simulink model "pvt_tegs_vienna"  (R2023b)
settings: Solver=ode14x  StartTime=0.0  StopTime=3*24*3600  FixedStep=1  RelTol=1e-06
PreLoadFcn:
  | sscv_hybrid_solar_panel_data
values from neighbouring files (symbols this model uses):
  Inclination = struct()    [meteo_data_struct.m]
  Irradiance_si = struct()    [meteo_data_struct.m]
  Irradiance_ts = struct()    [meteo_data_struct.m]
  load = struct()    [pvt_tegs_data.m]
  month = months{m}    [AUTOMATICO_mix.m]    (also in AUTOMATICO_parallel.m; AUTOMATICO_series.m)
  panel = struct()    [pvt_tegs_data.m]
  pipe = struct()    [pvt_tegs_data.m]
  pumps = struct()    [pvt_tegs_data.m]
  T_ext = struct()    [meteo_data_struct.m]
  tank = struct()    [pvt_tegs_data.m]
  teg = struct()    [pvt_tegs_data.m]
libraries: fl_lib x69, nesl_utility x35, simulink x5, ee_lib x2, My_second_lib x1, SimscapeFluids_lib x1
(part 2 of 2)

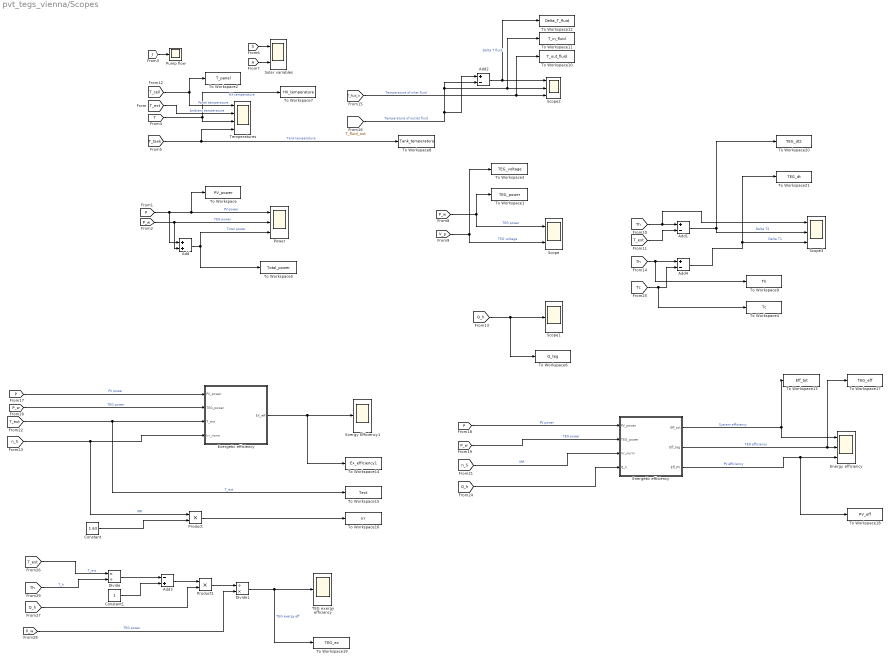
== system pvt_tegs_vienna/Scopes ==
  Add : Sum
  Add1 : Sum  Inputs=+-
  Add2 : Sum  Inputs=+-
  Add3 : Sum  Inputs=-+
  Add4 : Sum  Inputs=+-
  Constant : Constant  Value=1.63
  Constant1 : Constant
  Divide : Product  Inputs=*/
  Divide1 : Product  Inputs=/*
  Energetic efficiency : MATLAB Function  TreatAsAtomicUnit=on
  Energy efficiency : Scope  NumInputPorts=3
  Exergetic efficiency : MATLAB Function  TreatAsAtomicUnit=on
  Exergy Efficiency1 : Scope
  From7 : From  TagVisibility=global
  Power : Scope  NumInputPorts=3
  Product : Product
  Product1 : Product
  Pump flow : Scope
  Scope : Scope  NumInputPorts=2
  Scope1 : Scope
  Scope2 : Scope  NumInputPorts=3
  Scope3 : Scope  NumInputPorts=3
  Solar variables : Scope  NumInputPorts=2
  TEG exergy efficiency : Scope
  Temperatures : Scope  NumInputPorts=4
  To Workspace : ToWorkspace  VariableName=PV_power  SaveFormat=Structure With Time  SampleTime=-1
  To Workspace1 : ToWorkspace  VariableName=TEG_power  SaveFormat=Structure With Time  SampleTime=-1
  To Workspace10 : ToWorkspace  VariableName=T_out_fluid  SaveFormat=Structure With Time  SampleTime=-1
  To Workspace11 : ToWorkspace  VariableName=T_in_fluid  SaveFormat=Structure With Time  SampleTime=-1
  To Workspace12 : ToWorkspace  VariableName=Delta_T_fluid  SaveFormat=Structure With Time  SampleTime=-1
  To Workspace13 : ToWorkspace  VariableName=Eff_tot  SaveFormat=Structure With Time  SampleTime=-1
  To Workspace14 : ToWorkspace  VariableName=Ex_efficiency1  SaveFormat=Structure With Time  SampleTime=-1
  To Workspace15 : ToWorkspace  VariableName=Text  SaveFormat=Structure With Time  SampleTime=-1
  To Workspace16 : ToWorkspace  VariableName=Irr  SaveFormat=Structure With Time  SampleTime=-1
  To Workspace17 : ToWorkspace  VariableName=TEG_eff  SaveFormat=Structure With Time  SampleTime=-1
  To Workspace18 : ToWorkspace  VariableName=PV_eff  SaveFormat=Structure With Time  SampleTime=-1
  To Workspace19 : ToWorkspace  VariableName=TEG_ex  SaveFormat=Structure With Time  SampleTime=-1
  To Workspace2 : ToWorkspace  VariableName=T_panel  SaveFormat=Structure With Time  SampleTime=-1
  To Workspace20 : ToWorkspace  VariableName=TEG_dt2  SaveFormat=Structure With Time  SampleTime=-1
  To Workspace21 : ToWorkspace  VariableName=TEG_dt  SaveFormat=Structure With Time  SampleTime=-1
  To Workspace3 : ToWorkspace  VariableName=TEG_voltage  SaveFormat=Structure With Time  SampleTime=-1
  To Workspace4 : ToWorkspace  VariableName=Tc  SaveFormat=Structure With Time  SampleTime=-1
  To Workspace5 : ToWorkspace  VariableName=Total_power  SaveFormat=Structure With Time  SampleTime=-1
  To Workspace6 : ToWorkspace  VariableName=Q_teg  SaveFormat=Structure With Time  SampleTime=-1
  To Workspace7 : ToWorkspace  VariableName=HX_temperature  SaveFormat=Structure With Time  SampleTime=-1
  To Workspace8 : ToWorkspace  VariableName=Tank_temperature  SaveFormat=Structure With Time  SampleTime=-1
  To Workspace9 : ToWorkspace  VariableName=Th  SaveFormat=Structure With Time  SampleTime=-1
  wires:
  [P] -> Add/1, To Workspace/1, Power/1  "PV power"
  [J] -> Pump flow/1
  [S] -> Solar variables/1
  From7/1 -> Solar variables/2
  [T] -> To Workspace7/1, Temperatures/3  "HX temperature"
  [T_tank] -> Temperatures/4, To Workspace8/1  "Tank temperature"
  [T_ext] -> Temperatures/2  "Ambient temperature"
  [P_w] -> Add/2, Power/2  "TEG power"
  Add/1 -> To Workspace5/1, Power/3  "Total power"
  [P_w] -> To Workspace1/1, Scope/1  "TEG power"
  [V_p] -> To Workspace3/1, Scope/2  "TEG voltage"
  [T_cell] -> To Workspace2/1, Temperatures/1  "Panel temperature"
  [Q_h] -> To Workspace6/1, Scope1/1
  [T_fluid_out] -> Add2/1, To Workspace10/1, Scope2/3  "Temperature of outlet fluid"
  [T_fluid_in] -> To Workspace11/1, Scope2/2, Add2/2  "Temperature of inlet fluid"
  Add2/1 -> To Workspace12/1, Scope2/1  "Delta T fluid"
  [P] -> Exergetic efficiency/1(PV_power)  "PV power"
  [P_w] -> Exergetic efficiency/2(TEG_power)  "TEG power"
  [T_ext] -> To Workspace15/1, Exergetic efficiency/3(T_ext)  "T_ext"
  [n_S] -> Product/1, Exergetic efficiency/4(Irr_norm)  "IRR"
  Exergetic efficiency/1(EX_eff) -> To Workspace14/1, Exergy Efficiency1/1
  [P] -> Energetic efficiency/1(PV_power)  "PV power"
  [P_w] -> Energetic efficiency/2(TEG_power)  "TEG power"
  [n_S] -> Energetic efficiency/3(Irr_norm)  "IRR"
  [Q_h] -> Energetic efficiency/4(Q_h)
  Energetic efficiency/1(Eff_tot) -> To Workspace13/1, Energy efficiency/1  "System efficiency"
  Energetic efficiency/2(Eff_teg) -> Energy efficiency/2, To Workspace17/1  "TEG efficiency"
  Energetic efficiency/3(Eff_PV) -> To Workspace18/1, Energy efficiency/3  "PV efficiency"
  Constant/1 -> Product/2
  Product/1 -> To Workspace16/1
  [T_ext] -> Divide/1  "T_ext"
  Divide/1 -> Add3/1
  Constant1/1 -> Add3/2
  Add3/1 -> Product1/1
  [Q_h] -> Product1/2
  Product1/1 -> Divide1/1
  [P_w] -> Divide1/2  "TEG power"
  Divide1/1 -> To Workspace19/1, TEG exergy efficiency/1  "TEG exergy eff"
  [Th] -> Divide/2  "T_h"
  [Th] -> Add4/1, To Workspace9/1
  [Tc] -> To Workspace4/1, Add4/2
  Add4/1 -> To Workspace21/1, Scope3/3  "Delta T1"
  [Th] -> Scope3/1, Add1/1
  [T_ext] -> Add1/2
  Add1/1 -> To Workspace20/1, Scope3/2  "Delta T2"

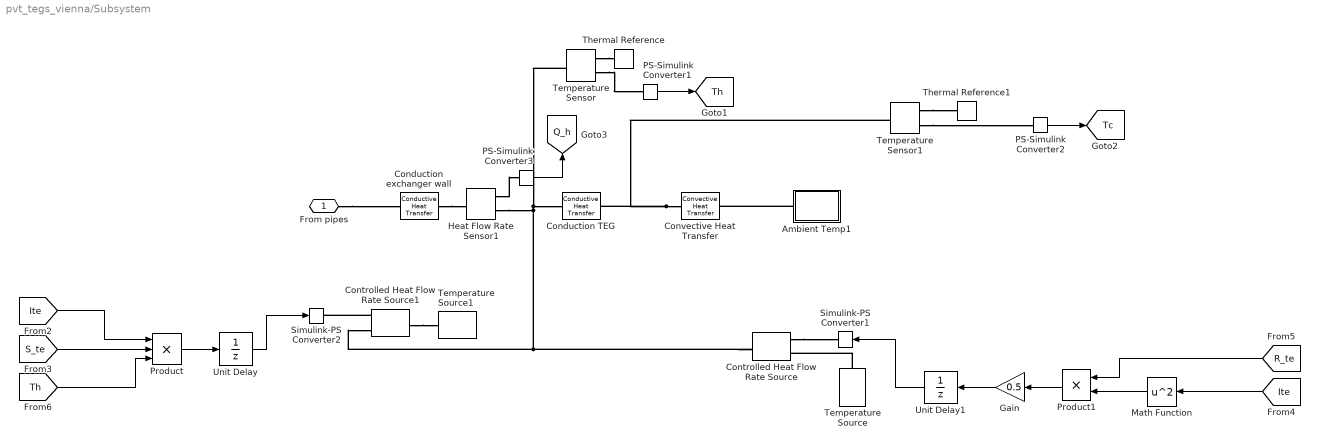
== system pvt_tegs_vienna/Subsystem ==
  Ambient Temp1 : Subsystem
  Conduction TEG : fl_lib/Thermal/Thermal Elements/Conductive Heat Transfer  thermal_type=foundation.enum.ConstantVariableTabulated.Constant  wall_geometry=foundation.enum.ConductionWallGeometry.Planar  area=teg.A_tot m^2  thickness=teg.d m  d_in=0.05 m  d_out=0.1 m  L=1 m  th_cond_min=10 W/(K*m)  th_cond=teg.l W/(m*K)  th_cond_TLU=[413, 401, 392, 383, 371, 357, 342] W/(K*m)  temp_TLU=[200, 273, 400, 600, 800, 1000, 1200] K  T_specify=off  T_priority=None  T=0 K  T_nominal_specify=off  T_nominal_unit=K  T_nominal_value=1  Q_specify=off  Q_priority=None  Q=0 W  Q_nominal_specify=off  Q_nominal_unit=W  Q_nominal_value=1
  Conduction exchanger wall : fl_lib/Thermal/Thermal Elements/Conductive Heat Transfer  thermal_type=foundation.enum.ConstantVariableTabulated.Constant  wall_geometry=foundation.enum.ConductionWallGeometry.Planar  area=teg.A_tot m^2  thickness=panel.heatTransfer.Le m  d_in=0.05 m  d_out=0.1 m  L=1 m  th_cond_min=10 W/(K*m)  th_cond=panel.heatTransfer.ke W/(m*K)  th_cond_TLU=[413, 401, 392, 383, 371, 357, 342] W/(K*m)  temp_TLU=[200, 273, 400, 600, 800, 1000, 1200] K  T_specify=off  T_priority=None  T=0 K  T_nominal_specify=off  T_nominal_unit=K  T_nominal_value=1  Q_specify=off  Q_priority=None  Q=0 W  Q_nominal_specify=off  Q_nominal_unit=W  Q_nominal_value=1
  Controlled Heat Flow Rate Source : fl_lib/Thermal/Thermal Sources/Controlled Heat Flow Rate Source
  Controlled Heat Flow Rate Source1 : fl_lib/Thermal/Thermal Sources/Controlled Heat Flow Rate Source
  Convective Heat Transfer : fl_lib/Thermal/Thermal Elements/Convective Heat Transfer  thermal_type=foundation.enum.constant_variable.constant  area=teg.A_tot m^2  heat_tr_coeff=teg.heat_conv W/(K*m^2)  min_heat_tr_coeff=1e-3 W/(K*m^2)  T_specify=off  T_priority=None  T=0 K  T_nominal_specify=off  T_nominal_unit=K  T_nominal_value=1  Q_specify=off  Q_priority=None  Q=0 W  Q_nominal_specify=off  Q_nominal_unit=W  Q_nominal_value=1
  Gain : Gain  Gain=0.5
  Heat Flow Rate Sensor1 : fl_lib/Thermal/Thermal Sensors/Heat Flow Rate Sensor
  Math Function : Math  Operator=square
  PS-Simulink Converter1 : nesl_utility/PS-Simulink Converter  PhysicalDomain=network_engine_domain  SubClassName=ps_output  LeftPortType=input  RightPortType=output  PseudoPeriodic=off  Frequencies=[]  VectorFormat=inherit  Unit=K  AffineConversion=off
  PS-Simulink Converter2 : nesl_utility/PS-Simulink Converter  PhysicalDomain=network_engine_domain  SubClassName=ps_output  LeftPortType=input  RightPortType=output  PseudoPeriodic=off  Frequencies=[]  VectorFormat=inherit  Unit=K  AffineConversion=off
  PS-Simulink Converter3 : nesl_utility/PS-Simulink Converter  PhysicalDomain=network_engine_domain  SubClassName=ps_output  LeftPortType=input  RightPortType=output  PseudoPeriodic=off  Frequencies=[]  VectorFormat=inherit  Unit=inherit  AffineConversion=off
  Product : Product  Inputs=3
  Product1 : Product
  Simulink-PS Converter1 : nesl_utility/Simulink-PS Converter  PhysicalDomain=network_engine_domain  SubClassName=ps_input  LeftPortType=input  RightPortType=output  PseudoPeriodic=off  Frequencies=[]  NoiseDistribution=none  NoiseParameters=[]  Unit=1  AffineConversion=off  FilteringAndDerivatives=provide  SimscapeFilterOrder=1  InputFilterTimeConstant=0.001  UdotUserProvided=0
  Simulink-PS Converter2 : nesl_utility/Simulink-PS Converter  PhysicalDomain=network_engine_domain  SubClassName=ps_input  LeftPortType=input  RightPortType=output  PseudoPeriodic=off  Frequencies=[]  NoiseDistribution=none  NoiseParameters=[]  Unit=1  AffineConversion=off  FilteringAndDerivatives=provide  SimscapeFilterOrder=1  InputFilterTimeConstant=0.001  UdotUserProvided=0
  Temperature Sensor : fl_lib/Thermal/Thermal Sensors/Temperature Sensor  temperature_measure=foundation.enum.MeasurementReference.difference
  Temperature Sensor1 : fl_lib/Thermal/Thermal Sensors/Temperature Sensor  temperature_measure=foundation.enum.MeasurementReference.difference
  Temperature Source : fl_lib/Thermal/Thermal Sources/Temperature Source  temperature=293.15 K
  Temperature Source1 : fl_lib/Thermal/Thermal Sources/Temperature Source  temperature=293.15 K
  Thermal Reference : fl_lib/Thermal/Thermal Elements/Thermal Reference
  Thermal Reference1 : fl_lib/Thermal/Thermal Elements/Thermal Reference
  Unit Delay : UnitDelay  SampleTime=-1  HasFrameUpgradeWarning=on
  Unit Delay1 : UnitDelay  SampleTime=-1  HasFrameUpgradeWarning=on
  From pipes : PMIOPort  Side=Right
  tag scope: Q_h=global, Tc=global, Th=global
  wires:
  PS-Simulink Converter1/1 -> [Th]
  [Ite] -> Math Function/1
  Math Function/1 -> Product1/2
  Product1/1 -> Gain/1
  [R_te] -> Product1/1
  [Ite] -> Product/1
  [S_te] -> Product/2
  Product/1 -> Unit Delay/1
  PS-Simulink Converter2/1 -> [Tc]
  [Th] -> Product/3
  Gain/1 -> Unit Delay1/1
  Unit Delay1/1 -> Simulink-PS Converter1/1
  Unit Delay/1 -> Simulink-PS Converter2/1
  PS-Simulink Converter3/1 -> [Q_h]
  connections:
  From pipes/RConn1 -- Conduction exchanger wall/LConn1
  Convective Heat Transfer/LConn1 -- Temperature Sensor1/LConn1 -- Conduction TEG/RConn1
  Ambient Temp1/LConn1 -- Convective Heat Transfer/RConn1
  Controlled Heat Flow Rate Source/LConn1 -- Temperature Sensor/LConn1 -- Conduction TEG/LConn1 -- Heat Flow Rate Sensor1/RConn2 -- Controlled Heat Flow Rate Source1/RConn2
  Temperature Sensor/RConn2 -- PS-Simulink Converter1/LConn1
  Temperature Sensor/RConn1 -- Thermal Reference/LConn1
  Temperature Source/LConn1 -- Controlled Heat Flow Rate Source/RConn2
  Controlled Heat Flow Rate Source/RConn1 -- Simulink-PS Converter1/RConn1
  Controlled Heat Flow Rate Source1/LConn1 -- Temperature Source1/LConn1
  Controlled Heat Flow Rate Source1/RConn1 -- Simulink-PS Converter2/RConn1
  Temperature Sensor1/RConn1 -- Thermal Reference1/LConn1
  Temperature Sensor1/RConn2 -- PS-Simulink Converter2/LConn1
  Conduction exchanger wall/RConn1 -- Heat Flow Rate Sensor1/LConn1
  Heat Flow Rate Sensor1/RConn1 -- PS-Simulink Converter3/LConn1

== system pvt_tegs_vienna/T sensor ==
  PS-Simulink Converter2 : nesl_utility/PS-Simulink Converter  PhysicalDomain=network_engine_domain  SubClassName=ps_output  LeftPortType=input  RightPortType=output  PseudoPeriodic=off  Frequencies=[]  VectorFormat=1-D array  Unit=K  AffineConversion=off
  Temperature Sensor : fl_lib/Thermal/Thermal Sensors/Temperature Sensor  temperature_measure=foundation.enum.MeasurementReference.difference
  Thermal Reference : fl_lib/Thermal/Thermal Elements/Thermal Reference
  A : PMIOPort  Side=Left
  tag scope: T=global
  wires:
  PS-Simulink Converter2/1 -> [T]
  connections:
  Temperature Sensor/LConn1 -- A/RConn1
  Thermal Reference/LConn1 -- Temperature Sensor/RConn1
  PS-Simulink Converter2/LConn1 -- Temperature Sensor/RConn2

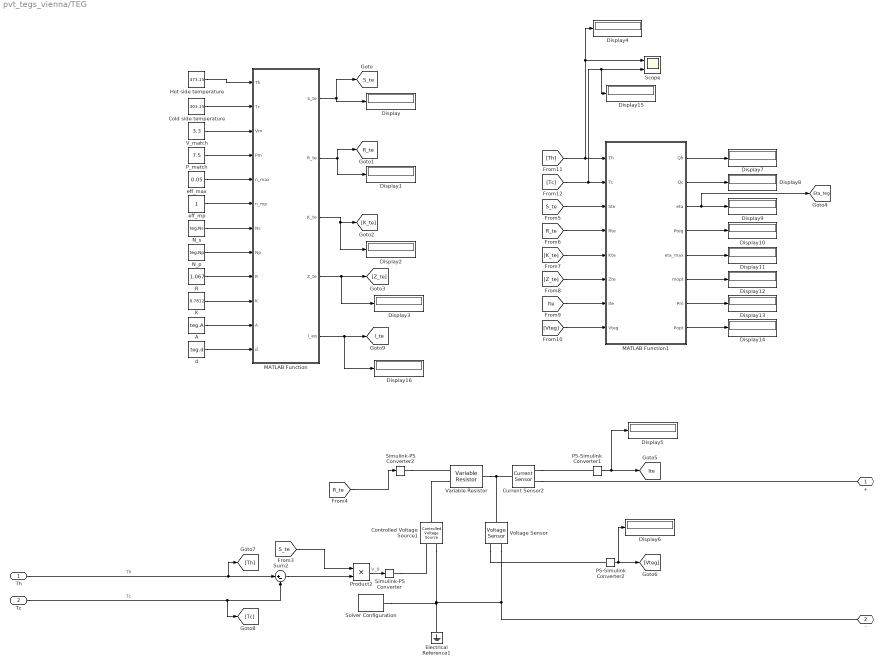
== system pvt_tegs_vienna/TEG ==
  Th : Inport
  Tc : Inport  Port=2
  A : Constant  Value=teg.A
  Cold side temperature : Constant  Value=303.15
  Controlled Voltage Source1 : fl_lib/Electrical/Electrical Sources/Controlled Voltage Source
  Current Sensor2 : fl_lib/Electrical/Electrical Sensors/Current Sensor
  Display{,1..16} (17 alike) : Display
  Electrical Reference1 : fl_lib/Electrical/Electrical Elements/Electrical Reference
  Hot side temperature : Constant  Value=473.15
  K : Constant  Value=0.7812
  MATLAB Function : MATLAB Function  TreatAsAtomicUnit=on
  MATLAB Function1 : MATLAB Function  TreatAsAtomicUnit=on
  N_p : Constant  Value=teg.Np
  N_s : Constant  Value=teg.Ns
  PS-Simulink Converter1 : nesl_utility/PS-Simulink Converter  PhysicalDomain=network_engine_domain  SubClassName=ps_output  LeftPortType=input  RightPortType=output  PseudoPeriodic=off  Frequencies=[]  VectorFormat=inherit  Unit=inherit  AffineConversion=off
  PS-Simulink Converter2 : nesl_utility/PS-Simulink Converter  PhysicalDomain=network_engine_domain  SubClassName=ps_output  LeftPortType=input  RightPortType=output  PseudoPeriodic=off  Frequencies=[]  VectorFormat=inherit  Unit=inherit  AffineConversion=off
  P_match : Constant  Value=7.5
  Product2 : Product
  R : Constant  Value=1.067
  Scope : Scope  NumInputPorts=2
  Simulink-PS Converter : nesl_utility/Simulink-PS Converter  PhysicalDomain=network_engine_domain  SubClassName=ps_input  LeftPortType=input  RightPortType=output  PseudoPeriodic=off  Frequencies=[]  NoiseDistribution=none  NoiseParameters=[]  Unit=1  AffineConversion=off  FilteringAndDerivatives=provide  SimscapeFilterOrder=1  InputFilterTimeConstant=0.001  UdotUserProvided=0
  Simulink-PS Converter2 : nesl_utility/Simulink-PS Converter  PhysicalDomain=network_engine_domain  SubClassName=ps_input  LeftPortType=input  RightPortType=output  PseudoPeriodic=off  Frequencies=[]  NoiseDistribution=none  NoiseParameters=[]  Unit=1  AffineConversion=off  FilteringAndDerivatives=provide  SimscapeFilterOrder=1  InputFilterTimeConstant=0.001  UdotUserProvided=0
  Solver Configuration : nesl_utility/Solver Configuration  PhysicalDomain=network_engine_domain  SubClassName=solver  LeftPortType=input  RightPortType=generic  Tones=[]  Harmonics=[]  SimulateNoise=off  Profile=off  UseLocalSampling=off  EnableSwitchedLinearOptims=on  FrequencyDomain=off  UseCCode=off  RelTol=0.001  AbsTol=0.001  MinStep=1e-09  ToWorkspace=off  RevertToSquareIcSolve=off  NumHomotopyIterations=100  PhasorMode=off  PhasorModeNumHarmonics=1  ConsistencySolver=NEWTON_XTOL_AFTER_FTOL  IndexReductionMethod=DerivativeReplacement  DoDC=off  ResidualTolerance=1e-09  ConsistencyTolSource=GLOBAL  ConsistencyAbsTol=0.001  ConsistencyRelTol=0.001  ConsistencyTolFactor=0.001  UseLocalSolver=off  LocalSolverChoice=NE_BACKWARD_EULER_ADVANCER  ResolveIndetEquations=on  FunctionEvalNumThread=1  LocalSolverSampleTime=0.001  DoFixedCost=off  MaxNonlinIter=3  MaxModeIter=2  ComputeImpulses=off  ImpulseIterations=2  LinearAlgebra=auto  LinearAlgebraNumThread=0  EquationFormulation=NE_TIME_EF  DelaysMemoryBudget=1024  AutomaticFiltering=on  FilteringTimeConstant=0.001  PartitionStorageMethod=AS_NEEDED  PartitionMemoryBudget=1024  PartitionMethod=ROBUST  MultibodyUseLocalSolver=off  MultibodyLocalSolverChoice=ODE1  MultibodyLocalSolverSampleTime=0.001
  Sum2 : Sum  Inputs=|+-
  V_match : Constant  Value=3.3
  Variable Resistor : fl_lib/Electrical/Electrical Elements/Variable Resistor  Rmin=0 Ohm  thermalEnable=false  thermal_mass=1 J/K  i_specify=off  i_priority=None  i=0 A  i_nominal_specify=off  i_nominal_unit=A  i_nominal_value=1  v_specify=off  v_priority=None  v=0 V  v_nominal_specify=off  v_nominal_unit=V  v_nominal_value=1  T_specify=off  T_priority=None  T=300 K  T_nominal_specify=off  T_nominal_unit=K  T_nominal_value=1
  Voltage Sensor : fl_lib/Electrical/Electrical Sensors/Voltage Sensor
  d : Constant  Value=teg.d
  eff_max : Constant  Value=0.05
  eff_mp : Constant
  + : PMIOPort  Side=Right
  - : PMIOPort  Port=2  Side=Right
  tag scope: Eta_teg=global, Ite=global, R_te=global, S_te=global, l_te=global
  wires:
  Th/1 -> [Th], Sum2/1  "Th"
  MATLAB Function/4(Z_te) -> Display3/1, [Z_te]
  [Z_te] -> MATLAB Function1/6(Zte)
  N_p/1 -> MATLAB Function/8(Np)
  eff_mp/1 -> MATLAB Function/6(n_mp)
  MATLAB Function/2(R_te) -> Display1/1, [R_te]
  eff_max/1 -> MATLAB Function/5(n_max)
  P_match/1 -> MATLAB Function/4(Pm)
  [Th] -> Display4/1, Scope/1, MATLAB Function1/1(Th)
  PS-Simulink Converter1/1 -> [Ite], Display5/1
  MATLAB Function1/1(Qh) -> Display7/1
  MATLAB Function/3(K_te) -> Display2/1, [K_te]
  [K_te] -> MATLAB Function1/5(Kte)
  PS-Simulink Converter2/1 -> Display6/1, [Vteg]
  MATLAB Function1/7(Pm) -> Display13/1
  Cold side temperature/1 -> MATLAB Function/2(Tc)
  MATLAB Function1/3(eta) -> [Eta_teg], Display9/1
  Tc/1 -> [Tc], Sum2/2  "Tc"
  Hot side temperature/1 -> MATLAB Function/1(Th)
  MATLAB Function/1(S_te) -> Display/1, [S_te]
  MATLAB Function1/6(mopt) -> Display12/1
  V_match/1 -> MATLAB Function/3(Vm)
  Product2/1 -> Simulink-PS Converter/1  "V_0"
  [S_te] -> Product2/1
  MATLAB Function1/4(Pteg) -> Display10/1
  N_s/1 -> MATLAB Function/7(Ns)
  [S_te] -> MATLAB Function1/3(Ste)
  MATLAB Function1/8(Popt) -> Display14/1
  MATLAB Function1/2(Qc) -> Display8/1
  [R_te] -> Simulink-PS Converter2/1
  MATLAB Function1/5(eta_max) -> Display11/1
  [Vteg] -> MATLAB Function1/8(Vteg)
  Sum2/1 -> Product2/2
  [R_te] -> MATLAB Function1/4(Rte)
  [Ite] -> MATLAB Function1/7(Ite)
  R/1 -> MATLAB Function/9(R)
  K/1 -> MATLAB Function/10(K)
  A/1 -> MATLAB Function/11(A)
  d/1 -> MATLAB Function/12(d)
  MATLAB Function/5(l_eq) -> Display16/1, [l_te]
  [Tc] -> Display15/1, Scope/2, MATLAB Function1/2(Tc)
  connections:
  Variable Resistor/RConn1 -- Voltage Sensor/LConn1 -- Current Sensor2/LConn1
  Current Sensor2/RConn2 -- +/RConn1
  Current Sensor2/RConn1 -- PS-Simulink Converter1/LConn1
  Controlled Voltage Source1/RConn2 -- Solver Configuration/RConn1 -- Electrical Reference1/LConn1 -- -/RConn1 -- Voltage Sensor/RConn2
  Controlled Voltage Source1/LConn1 -- Variable Resistor/LConn2
  Simulink-PS Converter/RConn1 -- Controlled Voltage Source1/RConn1
  Simulink-PS Converter2/RConn1 -- Variable Resistor/LConn1
  Voltage Sensor/RConn1 -- PS-Simulink Converter2/LConn1

== system pvt_tegs_vienna/Subsystem/Ambient Temp1 ==
  Controlled Temperature Source : fl_lib/Thermal/Thermal Sources/Controlled Temperature Source
  Simulink-PS Converter1 : nesl_utility/Simulink-PS Converter  PhysicalDomain=network_engine_domain  SubClassName=ps_input  LeftPortType=input  RightPortType=output  PseudoPeriodic=off  Frequencies=[]  NoiseDistribution=none  NoiseParameters=[]  Unit=K  AffineConversion=off  FilteringAndDerivatives=provide  SimscapeFilterOrder=1  InputFilterTimeConstant=0.001  UdotUserProvided=0
  Thermal Reference1 : fl_lib/Thermal/Thermal Elements/Thermal Reference
  Conn1 : PMIOPort  Side=Left
  wires:
  [T_ext] -> Simulink-PS Converter1/1
  connections:
  Controlled Temperature Source/LConn1 -- Conn1/RConn1
  Thermal Reference1/LConn1 -- Controlled Temperature Source/RConn2
  Simulink-PS Converter1/RConn1 -- Controlled Temperature Source/RConn1

== matlab function pvt_tegs_vienna/TEG/MATLAB Function ==
  data: Th input; S_te output; Tc input; Vm input; Pm input; n_max input; n_mp input; Ns input; Np input; R_te output; K_te output; Z_te output; R input; K input; l_eq output; A input; d input
function [S_te, R_te, K_te, Z_te, l_eq] = Teg_properties(Th,Tc,Vm,Pm,n_max,n_mp,Ns,Np,R,K,A,d)

%MODULE:
%Th: hot side temperature at which TEG properties are measured
%Tc: cold side temperature at which TEG properties are measured
%Vm: matched load voltage of module (maximum power at given DT)
%Pm: matched power (maximum power at given DT)
%n_max: maximum efficiency of TEG at given DT
%n_mp: matched efficiency (efficiency of TEG at maximum power point g.DT)
%A: area of the module [m^2]
%d: thickness of the module [m]

%CONNECTION:
%Ns: number of series-connected TEGs modules
%Np: number of electrically parallel connected groups of modules. 

%Temperature difference
D_T=Th-Tc;

%Average temperature
T_avr=(Th+Tc)/2;

%Seebeck coefficient of module
Sm=2*Vm/D_T;

%Internal resistance of module
if isnan(R) 
    Rm=Vm^2/Pm;
else
    Rm=R;
end

%Conduttance of the module
if isnan(K)
    Km=(Sm^2*(D_T-n_max*Th)^2)/(2*(2-n_max)*D_T*n_max*Rm);
else
    Km=K;
end

%Km=(Sm^2*(D_T-n_mp*(Th+T_avr)))/(4*n_mp*Rm)


%Figure of merit of module
Zm=Sm^2/(Rm*Km);

%Converting the parameters for 1 module to Ns, Np modules
S_te=Ns*Sm;
R_te=(Ns/Np)*Rm;
K_te=Ns*Np*Km;
Z_te=Zm;
l_eq=(d*K_te)/A;
end

== matlab function pvt_tegs_vienna/Optical model/MATLAB Function ==
  data: S input; Ir output; Incl input; heatg output; powAbspv output; panel parameter
function [Ir, heatg, powAbspv] = optics(S, Incl, panel)
    
    %This function computes the reflection, absorption and transmission in
    %the glass to compute the irradiation to the PV cells, the heat absorbed 
    %in the glass and the radiation power absorbed in the PV cells,
    %it is based on Fresnel's laws, depending on the incident angle
    
    Ncell = panel.geometry.Ncell;
    Acell = panel.geometry.Acell;
    Apanel = panel.geometry.Apanel;
    ng = panel.optical.ng;
    absg = panel.optical.absg;
    dg = panel.optical.dg;
    rpv = panel.optical.rpv;
   

    % Fresnel equations 1st boundary
    r1p =  ( ng^2*cos(Incl) - sqrt(ng^2 - sin(Incl)^2) )^2/( ng^2*cos(Incl) + sqrt( ng^2 - sin(Incl)^2 ) )^2; %P polarization
    r1s =  ( cos(Incl) - sqrt(ng^2 - sin(Incl)^2) )^2/( cos(Incl) + sqrt( ng^2 - sin(Incl)^2 ) )^2; %S polarization
    r1 = 0.5*(r1p + r1s); %Effective reflectance
    t1 = 1-r1;

    nga = 1/ng; %refractive index glass -> air
    th2 = asin(sin(Incl)/ng);  %Snell's law to compute angle of incidence on 2nd boundary

    % Fresnel equations 2nd boundary
    r2p = ( nga^2*cos(th2) - sqrt(nga^2 - sin(th2)^2) )^2/( nga^2*cos(th2) + sqrt( nga^2 - sin(th2)^2 ) )^2 ;
    r2s = ( cos(th2) - sqrt(nga^2 - sin(th2)^2) )^2/( cos(th2) + sqrt( nga^2 - sin(th2)^2 ) )^2 ;
    r2 = 0.5*(r2p + r2s); %Effective reflectance
    t2 = 1 - r2;

    taug = exp(-absg*dg/cos(th2)); 
    
    %Total coefficients for infinite reflections between 2 parallel boundaries
    Transg = t1*taug*t2/(1 - r1*r2*taug^2);
    Reflg = r1 + (t1^2*taug^2*r2)/(1 - r1*r2*taug^2);
    Absg = 1 - Transg - Reflg; 

    Ir = S*Transg; %Irradiation to the PV cells
    heatg = Apanel*Absg*S; %heat absorbed in the glass
    powAbspv = Apanel*Transg*(1-rpv)*S; %radiation power absorbed by PV cells. Part of it transforms in electrical power
    
end

== matlab function pvt_tegs_vienna/TEG/MATLAB Function1 ==
  data: Th input; Qh output; Tc input; Ste input; Rte input; Kte input; Zte input; Ite input; Vteg input; Qc output; eta output; Pteg output; eta_max output; mopt output; Pm output; Popt output
function [Qh,Qc,eta,Pteg,eta_max,mopt,Pm,Popt] = TEG_operation(Th,Tc,Ste,Rte,Kte,Zte,Ite,Vteg)

%Average temperature 
Tavr=(Th+Tc)/2;

%Qh: absorbed heat from hot side [W]
Qh=Ste*Ite*Th + Kte*(Th-Tc) - (Ite^2)*(Rte/2);

%Qc: emitted heat from the cold side to the environment [W]
Qc=Ste*Ite*Tc + Kte*(Th-Tc) + (Ite^2)*(Rte/2);

%Pteg: generated electrical output power [W] --> Pteg = Qh-Qc
Pteg=Vteg*Ite;

%eta: efficiency of thermoelectric generator [-]
eta=Pteg/Qh;

%eta_max: maximum efficiency achievable by the TEG at Th and Tc [-]
eta_max=(1-(Tc/Th))*(sqrt(complex(1+Zte*Tavr))-1)/(sqrt(complex(1+Zte*Tavr))+(Tc/Th));

%mopt: optimal load ratio (maximized the efficiency) assuming a resistive
%load (m=Rl/Rte) [-]
mopt=sqrt(1+Zte*Tavr);

%Pm: matched power of TEG i.e maximum power achievable at given Th and Tc
%[W]
Pm=(Ste^2*(Th-Tc)^2)/4*Rte;

%Popt: power output of TEG under eta_max condition, assumung a resistive
%load [W]
Popt=(Ste^2*(Th-Tc)^2*mopt)/(Rte*(mopt+1)^2);

end

== matlab function pvt_tegs_vienna/Scopes/Exergetic efficiency ==
  data: PV_power input; EX_eff output; TEG_power input; T_ext input; Irr_norm input
function EX_eff  = EX_eff(PV_power, TEG_power, T_ext, Irr_norm)

%Sun temperature [K]
T_sun = 5777; 

%Pump consumption [W]
Pump_cons = 0.0284;

%Area panel [m^2]
A_panel = 1.6315; 


if Irr_norm > 10
    EX_eff = (PV_power + TEG_power - Pump_cons)/(Irr_norm*A_panel*(1-(4/3)*(T_ext/T_sun)+(1/3)*(T_ext/T_sun)^4));
else
    EX_eff = 0;
end

== matlab function pvt_tegs_vienna/Scopes/Energetic efficiency ==
  data: PV_power input; Eff_tot output; TEG_power input; Irr_norm input; Q_h input; Eff_teg output; Eff_PV output
function [Eff_tot, Eff_teg, Eff_PV]  = En_eff(PV_power, TEG_power, Irr_norm, Q_h)

%Sun temperature [K]
T_sun = 5777; 

%Pump consumption [W]
Pump_cons = 0.0284;

%Area panel [m^2]
A_panel = 1.6315; 

%PV/T-TEGs efficiency

if Irr_norm > 10
    Eff_tot = (PV_power + TEG_power - Pump_cons)/(Irr_norm*A_panel);
else
    Eff_tot = 0;
end

% TEG system efficiency

Eff_teg = TEG_power/Q_h;

%PV panel efficiency

Eff_PV = PV_power/(A_panel*Irr_norm);

== matlab function pvt_tegs_vienna/Converter & Load1/MATLAB Function2 ==
  data: input input; y output; prevState input
function y = hysteresis(input, prevState)
    % Logica di isteresi
    if input > 0.03
        y = 2;
    elseif input < 0.01
        y = 0;
    else
        y = prevState; % Mantieni lo stato precedente
    end
end
